simulink model "Day06"  (R2024b)
settings: Solver=VariableStepAuto  StartTime=0.0  StopTime=10.0  RelTol=1e-3
libraries: simulink x2
settings Model: Creator=jun_mac  LastModifiedBy=jun_mac

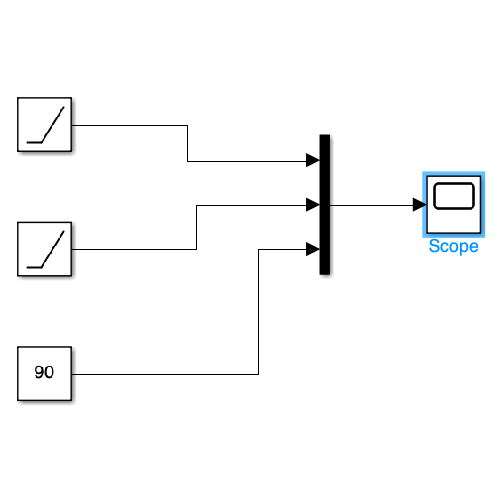
[thumbnail: Simulink's stored preview of the top-level diagram]
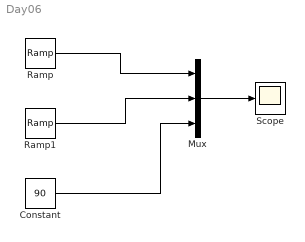
== system Day06 ==
  Constant : Constant  Value=90
  Mux : Mux  Inputs=3
  Ramp : simulink/Sources/Ramp  slope=12  start=0  InitialOutput=0
  Ramp1 : simulink/Sources/Ramp  slope=250  start=0  InitialOutput=0
  Scope : Scope
  wires:
  Ramp/1 -> Mux/1
  Mux/1 -> Scope/1
  Ramp1/1 -> Mux/2
  Constant/1 -> Mux/3
